simulink model "OpenLoopSimulation"  (R2022a)
settings: Solver=ode4  StartTime=0.0  StopTime=100  FixedStep=0.1  RelTol=1e-3
settings Model: Creator=Jan-Robin  LastModifiedBy=Jan-Robin

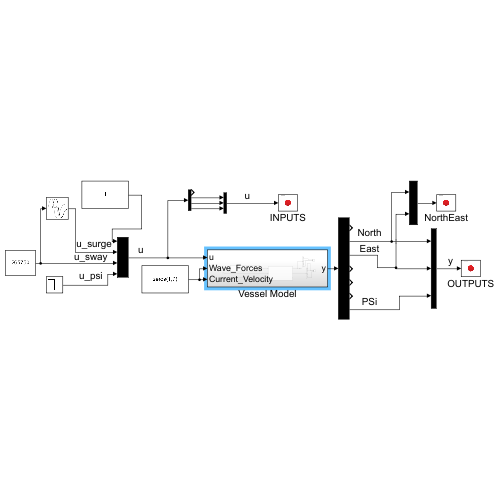
[thumbnail: Simulink's stored preview of the top-level diagram]
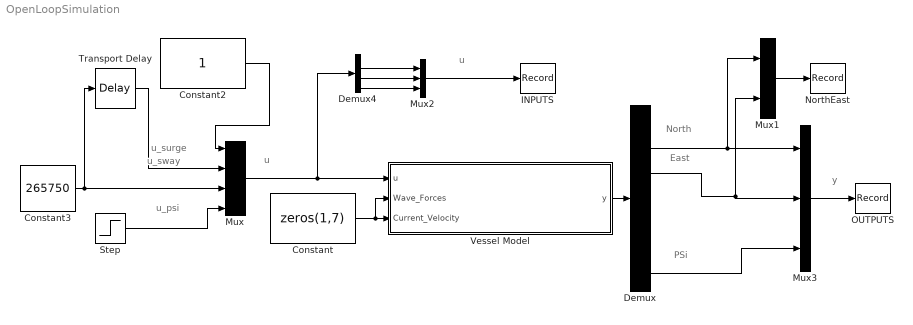
== system OpenLoopSimulation ==
  note: u_psi
  note: u_sway
  note: u_surge
  note: y
  note: u
  note: North
  note: PSi
  note: East
  note: u
  Constant : Constant  Value=zeros(1,7)
  Constant2 : Constant
  Constant3 : Constant  Value=265750
  Demux : Demux  Outputs=7
  Demux4 : Demux
  INPUTS : Record  VariableName=INPUT  RecordToWorkspace=on  FileSettingsInternal="{\"entries\":[{\"content\":{\"excelSettings\":{\"content\":{},\"type\":\"Streamout.ExcelSettings\"}},\"type\":\"Streamout.FileSettingStorage\",\"uuid\":\"\"}],\"packageUris\":[\"http:\\/\\/schema.mathworks.com\\/mf0\\/streamout_blocks\\/R2020a\"],\"version\":\"1.0\"}"  SignalsInternal="{\"entries\":[{\"content\":{\"signals\":[{\"content\":{\"blockPath\":[],\"channel\":[],\"dimensions\":[3],\"domain\":\"\",\"hasChildren\":true,\"lineColor\":\"#139fff\",\"plots\":[],\"port\":1,\"sid\":[\"\"],\"signalID\":1352,\"signalName\":\"Mux2\"},\"type\":\"RecordBlkView.Signal\",\"uuid\":\"\"},{\"content\":{\"blockPath\":[],\"channel\":[1],\"dimensions\":[3],\"domain\":\"\",\"lineColor\":\"#64d413\",\"parentID\":1352,\"plots\":[1],\"port\":1,\"sid\":[\"\"],\"signalID\":1353,\"signalName\":\"Mux2\"},\"type\":\"RecordBlkView.Signal\",\"uuid\":\"\"},{\"content\":{\"blockPath\":[],\"channel\":[2],\"dimensions\":[3],\"domain\":\"\",\"lineColor\":\"#22b573\",\"parentID\":1352,\"plots\":[1],\"port\":1,\"sid\":[\"\"],\"signalID\":1380,\"signalName\":\"Mux2\"},\"type\":\"RecordBlkView.Signal\",\"uuid\":\"\"},{\"content\":{\"blockPath\":[],\"channel\":[3],\"dimensions\":[3],\"domain\":\"\",\"lineColor\":\"#0072bd\",\"parentID\":1352,\"plots\":[1],\"port\":1,\"sid\":[\"\"],\"signalID\":1381,\"signalName\":\"Mux2\"},\"type\":\"RecordBlkView.Signal\",\"uuid\":\"\"}]},\"type\":\"RecordBlkView.InputSignals\",\"uuid\":\"\"}],\"packageUris\":[\"http:\\/\\/schema.mathworks.com\\/mf0\\/streamout_blocks\\/R2020a\"],\"version\":\"1.0\"}"  VisualizationBindings="{\"sparklinesplugin\":{\"info\":[{\"bindingParametersList\":[],\"subplotID\":1}]}}"
  Mux : Mux
  Mux1 : Mux  Inputs=2
  Mux2 : Mux  Inputs=3
  Mux3 : Mux  Inputs=3
  NorthEast : Record  VariableName=xydata  Filename=C:\Users\Jan-Robin\OneDrive - Troms og Finnmark fylkeskommune\Documents\Studie\Master\OSP\data.xlsx  RecordToWorkspace=on  RecordToFile=on  FileSettingsInternal="{\"entries\":[{\"content\":{\"excelSettings\":{\"content\":{},\"type\":\"Streamout.ExcelSettings\"}},\"type\":\"Streamout.FileSettingStorage\",\"uuid\":\"\"}],\"packageUris\":[\"http:\\/\\/schema.mathworks.com\\/mf0\\/streamout_blocks\\/R2020a\"],\"version\":\"1.0\"}"  Layout=[1 1]  SignalsInternal="{\"entries\":[{\"content\":{\"signals\":[{\"content\":{\"blockPath\":[],\"channel\":[],\"dimensions\":[2],\"domain\":\"\",\"hasChildren\":true,\"lineColor\":\"#b746ff\",\"plots\":[],\"port\":1,\"sid\":[\"\"],\"signalID\":1357,\"signalName\":\"Mux1\"},\"type\":\"RecordBlkView.Signal\",\"uuid\":\"\"},{\"content\":{\"blockPath\":[],\"channel\":[1],\"dimensions\":[2],\"domain\":\"\",\"lineColor\":\"#4dbeee\",\"parentID\":1357,\"plots\":[],\"port\":1,\"sid\":[\"\"],\"signalID\":1358,\"signalName\":\"Mux1\"},\"type\":\"RecordBlkView.Signal\",\"uuid\":\"\"},{\"content\":{\"blockPath\":[],\"channel\":[2],\"dimensions\":[2],\"domain\":\"\",\"lineColor\":\"#edb120\",\"parentID\":1357,\"plots\":[],\"port\":1,\"sid\":[\"\"],\"signalID\":1382,\"signalName\":\"Mux1\"},\"type\":\"RecordBlkView.Signal\",\"uuid\":\"\"}]},\"type\":\"RecordBlkView.InputSignals\",\"uuid\":\"\"}],\"packageUris\":[\"http:\\/\\/schema.mathworks.com\\/mf0\\/streamout_blocks\\/R2020a\"],\"version\":\"1.0\"}"  VisualizationBindings="{\"sparklinesplugin\":{\"info\":[{\"bindingParametersList\":[],\"subplotID\":1}]}}"
  OUTPUTS : Record  VariableName=OUTPUT  RecordToWorkspace=on  FileSettingsInternal="{\"entries\":[{\"content\":{\"excelSettings\":{\"content\":{},\"type\":\"Streamout.ExcelSettings\"}},\"type\":\"Streamout.FileSettingStorage\",\"uuid\":\"\"}],\"packageUris\":[\"http:\\/\\/schema.mathworks.com\\/mf0\\/streamout_blocks\\/R2020a\"],\"version\":\"1.0\"}"  Layout=[1 1]  SignalsInternal="{\"entries\":[{\"content\":{\"signals\":[{\"content\":{\"blockPath\":[],\"channel\":[],\"dimensions\":[3],\"domain\":\"\",\"hasChildren\":true,\"lineColor\":\"#ff13a6\",\"plots\":[],\"port\":1,\"sid\":[\"\"],\"signalID\":1362,\"signalName\":\"Mux3\"},\"type\":\"RecordBlkView.Signal\",\"uuid\":\"\"},{\"content\":{\"blockPath\":[],\"channel\":[1],\"dimensions\":[3],\"domain\":\"\",\"lineColor\":\"#a2142f\",\"parentID\":1362,\"plots\":[1],\"port\":1,\"sid\":[\"\"],\"signalID\":1363,\"signalName\":\"Mux3\"},\"type\":\"RecordBlkView.Signal\",\"uuid\":\"\"},{\"content\":{\"blockPath\":[],\"channel\":[2],\"dimensions\":[3],\"domain\":\"\",\"lineColor\":\"#edb120\",\"parentID\":1362,\"plots\":[1],\"port\":1,\"sid\":[\"\"],\"signalID\":1383,\"signalName\":\"Mux3\"},\"type\":\"RecordBlkView.Signal\",\"uuid\":\"\"},{\"content\":{\"blockPath\":[],\"channel\":[3],\"dimensions\":[3],\"domain\":\"\",\"lineColor\":\"#7e2f8e\",\"parentID\":1362,\"plots\":[1],\"port\":1,\"sid\":[\"\"],\"signalID\":1384,\"signalName\":\"Mux3\"},\"type\":\"RecordBlkView.Signal\",\"uuid\":\"\"}]},\"type\":\"RecordBlkView.InputSignals\",\"uuid\":\"\"}],\"packageUris\":[\"http:\\/\\/schema.mathworks.com\\/mf0\\/streamout_blocks\\/R2020a\"],\"version\":\"1.0\"}"  VisualizationBindings="{\"sparklinesplugin\":{\"info\":[{\"bindingParametersList\":[],\"subplotID\":1}]}}"
  Step : Step  Time=300  Before=265750  After=0  SampleTime=0
  Transport Delay : TransportDelay  DelayTime=10
  Vessel Model : Subsystem
  wires:
  Constant2/1 -> Mux/1
  Vessel Model/1(y) -> Demux/1
  Constant/1 -> Vessel Model/3(Current_Velocity), Vessel Model/2(Wave_Forces)
  Mux3/1 -> OUTPUTS/1
  Demux/7 -> Mux3/3
  Demux4/4 -> Mux2/3
  Mux2/1 -> INPUTS/1
  Demux4/2 -> Mux2/1
  Demux/3 -> Mux3/2, Mux1/2
  Demux4/3 -> Mux2/2
  Demux/2 -> Mux3/1, Mux1/1
  Mux/1 -> Demux4/1, Vessel Model/1(u)
  Constant3/1 -> Transport Delay/1, Mux/3
  Mux1/1 -> NorthEast/1
  Transport Delay/1 -> Mux/2
  Step/1 -> Mux/4

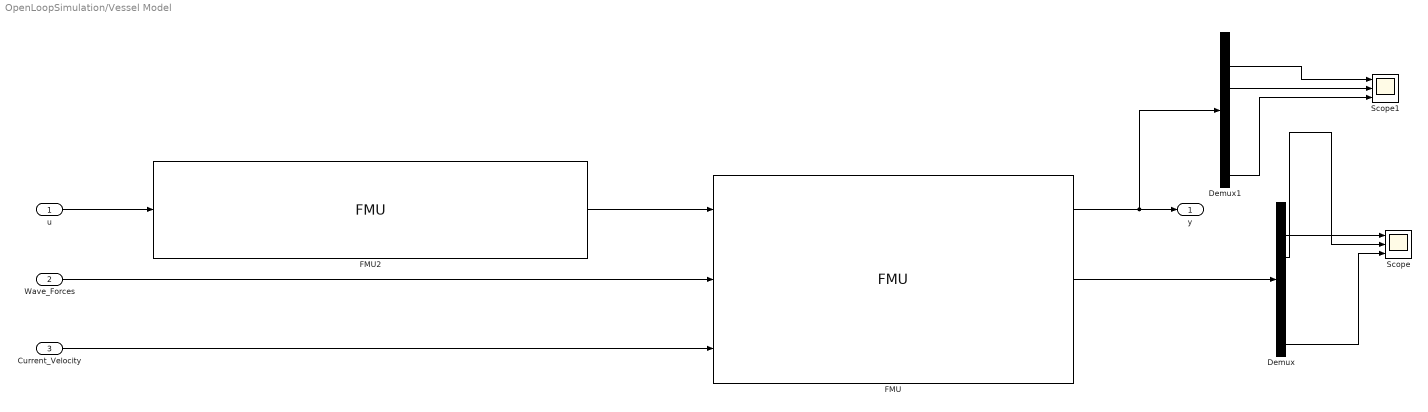
== system OpenLoopSimulation/Vessel Model ==
  u : Inport
  Wave_Forces : Inport  Port=2
  Current_Velocity : Inport  Port=3
  Demux : Demux  Outputs=7
  Demux1 : Demux  Outputs=7
  FMU : FMU  FMUName=VesselModel.fmu  FMUMode=CoSimulation  Axc=106.0  Ayc=419.0  Bv_0_=44000.0  Bv_1_=0.0  Bv_2_=0.0  Bv_3_=0.0  Bv_4_=0.0  Bv_5_=0.0  Bv_6_=0.0  Bv_7_=177000.0  Bv_8_=0.0  Bv_9_=0.0  Bv_10_=0.0  Bv_11_=0.0  Bv_12_=0.0  Bv_13_=0.0  Bv_14_=0.0  Bv_15_=0.0  Bv_16_=0.0  Bv_17_=0.0  Bv_18_=0.0  Bv_19_=0.0  Bv_20_=0.0  Bv_21_=686000.0  Bv_22_=0.0  Bv_23_=0.0  Bv_24_=0.0  Bv_25_=0.0  Bv_26_=0.0  Bv_27_=0.0  Bv_28_=0.0  Bv_29_=0.0  Bv_30_=0.0  Bv_31_=0.0  Bv_32_=0.0  Bv_33_=0.0  Bv_34_=0.0  Bv_35_=1.0259E+7  Cx=1.0  Cy=0.7812  Dp_0_=5300.0  Dp_1_=0.0  Dp_2_=0.0  Dp_3_=0.0  Dp_4_=0.0  Dp_5_=0.0  Dp_6_=0.0  Dp_7_=21100.0  Dp_8_=0.0  Dp_9_=-20300.0  Dp_10_=0.0  Dp_11_=294000.0  Dp_12_=0.0  Dp_13_=0.0  Dp_14_=1900.0  Dp_15_=0.0  Dp_16_=-68400.0  Dp_17_=0.0  Dp_18_=0.0  Dp_19_=-20300.0  Dp_20_=0.0  Dp_21_=7600.0  Dp_22_=0.0  Dp_23_=-201300.0  Dp_24_=0.0  Dp_25_=0.0  Dp_26_=-68400.0  Dp_27_=0.0  Dp_28_=819700.0  Dp_29_=0.0  Dp_30_=0.0  Dp_31_=294000.0  Dp_32_=0.0  Dp_33_=-201300.0  Dp_34_=0.0  Dp_35_=1.8944E+6  G_0_=0.0  G_1_=0.0  G_2_=0.0  G_3_=0.0  G_4_=0.0  G_5_=0.0  G_6_=0.0  G_7_=0.0  G_8_=0.0  G_9_=0.0  G_10_=0.0  G_11_=0.0  G_12_=0.0  G_13_=0.0  G_14_=2.44E+6  G_15_=0.0  G_16_=1.78E+6  G_17_=0.0  G_18_=0.0  G_19_=0.0  G_20_=0.0  G_21_=5.11E+6  G_22_=0.0  G_23_=0.0  G_24_=0.0  G_25_=0.0  G_26_=1.78E+6  G_27_=0.0  G_28_=1.2737E+8  G_29_=0.0  G_30_=0.0  G_31_=0.0  G_32_=0.0  G_33_=0.0  G_34_=0.0  G_35_=0.0  Lpp=28.9  Minv_0_=1.268E-6  Minv_1_=0.0  Minv_2_=0.0  Minv_3_=0.0  Minv_4_=0.0  Minv_5_=0.0  Minv_6_=0.0  Minv_7_=1.083E-6  Minv_8_=0.0  Minv_9_=1.2E-8  Minv_10_=0.0  Minv_11_=1.0E-9  Minv_12_=0.0  Minv_13_=0.0  Minv_14_=5.9200000000000011E-7  Minv_15_=0.0  Minv_16_=-1.3E-8  Minv_17_=0.0  Minv_18_=0.0  Minv_19_=1.2E-8  Minv_20_=0.0  Minv_21_=1.0000000000000001E-7  Minv_22_=0.0  Minv_23_=-1.0E-9  Minv_24_=0.0  Minv_25_=0.0  Minv_26_=-1.3E-8  Minv_27_=0.0  Minv_28_=1.2E-8  Minv_29_=0.0  Minv_30_=0.0  Minv_31_=1.0E-9  Minv_32_=0.0  Minv_33_=-1.0E-9  Minv_34_=0.0  Minv_35_=2.0E-8  N=20.0  X_DOF_DP_model_Integrator1__InitialCondition_0_=0.0  X_DOF_DP_model_Integrator1__InitialCondition_1_=0.0  X_DOF_DP_model_Integrator1__InitialCondition_2_=0.0  X_DOF_DP_model_Integrator1__InitialCondition_3_=0.0  X_DOF_DP_model_Integrator1__InitialCondition_4_=0.0  X_DOF_DP_model_Integrator1__InitialCondition_5_=0.0  X_DOF_DP_model_Integrator2_InitialCondition_0_=0.0  X_DOF_DP_model_Integrator2_InitialCondition_1_=0.0  X_DOF_DP_model_Integrator2_InitialCondition_2_=0.0  X_DOF_DP_model_Integrator2_InitialCondition_3_=0.0  X_DOF_DP_model_Integrator2_InitialCondition_4_=0.0  X_DOF_DP_model_Integrator2_InitialCondition_5_=0.0  X_DOF_DP_model_Rotate_yaw_T_Constant_Value=0.0  X_DOF_DP_model_Rotate_yaw_T_psi_Value=0.0  X_DOF_DP_model_X_DOF_transformation_Euler_angles_to_att=0.0  X_DOF_DP_model_X_DOF_transformation_Euler_angles_to_att_2=1.0  X_DOF_DP_model_zero_Value=0.0  rho=1025.0  mask(VesselModel [Co-Simulation, v2.0]){}
      mask Display:
      | disp('VesselModel');
      | port_label('output',1,'Vessel_Position');
      | port_label('output',2,'Vessel_Velocity');
      | port_label('output',3,'Vessel_Acceleration');
      | port_label('input',1,'Thrust');
      | port_label('input',2,'Wave_Forces');
      | port_label('input',3,'Current_Velocity');
  FMU2 : FMU  FMUName=ThrusterDynamics.fmu  FMUMode=CoSimulation  Heave_Thrust=struct('Value',0.0)  Merge1=struct('InitialOutput',0.0)  Pitch_Thrust=struct('Value',0.0)  Roll_Thrust=struct('Value',0.0)  Thruster_Dynamics=struct('Surge_Thrust_Dynamics',struct('A',-0.2,'C',0.2),'Sway_Thrust_Dynamics',struct('A',-0.2,'C',0.2),'Yaw_Thrust_Dynamics',struct('A',-0.2,'C',0.2))  enableDynamics=on  enableSaturation=on  maxThrust=[1.0E+10,1.0E+10,1.0E+11]  mask(ThrusterDynamics [Co-Simulation, v2.0]){}
      mask Display:
      | disp('ThrusterDynamics');
      | port_label('output',1,'Thrust');
      | port_label('input',1,'Commanded_Thrust');
  Scope : Scope  NumInputPorts=3
  Scope1 : Scope  NumInputPorts=3
  y : Outport
  wires:
  u/1 -> FMU2/1
  FMU2/1 -> FMU/1
  FMU/1 -> Demux1/1, y/1
  Wave_Forces/1 -> FMU/2
  Current_Velocity/1 -> FMU/3
  FMU/2 -> Demux/1
  Demux/2 -> Scope/1
  Demux/3 -> Scope/2
  Demux/7 -> Scope/3
  Demux1/2 -> Scope1/1
  Demux1/3 -> Scope1/2
  Demux1/7 -> Scope1/3
